simulink model "Flowchart6"  (Simulink 8.7)
settings: Solver=FixedStepDiscrete  StartTime=0.0  StopTime=10.0  RelTol=1e-3
settings Model: Creator=scaife  LastModifiedBy=bourbouh  ExtModeAutoUpdateStatusClock=off
settings DataIOCC: SignalLoggingSaveFormat=ModelDataLogs
settings OptimizationCC: InitFltsAndDblsToZero=on
settings DebuggingCC: SaveWithParameterizedLinksMsg=none  SignalResolutionControl=TryResolveAllWithWarning  SolverPrmCheckMsg=warning  MultiTaskDSMMsg=warning  MultiTaskCondExecSysMsg=none
settings SFSimCC: SimParseCustomCode=off
settings GRTTargetCC: TargetFcnLib=ansi_tfl_tmw.mat  GeneratePreprocessorConditionals=Use local settings  CombineOutputUpdateFcns=off  GRTInterface=on

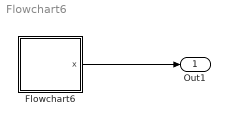
== system Flowchart6 ==
  Flowchart6 : Stateflow chart  TreatAsAtomicUnit=on
  Out1 : Outport
  wires:
  Flowchart6/1(x) -> Out1/1

== stateflow chart Flowchart6 ==
  state A
    (default) -> (junction 4)
    A -> (junction 4)
    (junction 4) -> (junction 5) : {x++;}
  data: x output int32
